simulink model "Aruduino_DCmoter_test"  (R2015a)
settings: Solver=ode3  StartTime=0.0  StopTime=10.0  RelTol=1e-3
libraries: arduinolib x5
settings Model: SimulationMode=external  ExtModeTrigDuration=2  Creator=Edwin Ri  LastModifiedBy=Edwin Ri
settings OptimizationCC: OptimizeModelRefInitCode=on  LifeSpan=1
settings DebuggingCC: UnderspecifiedInitializationDetection=Classic  MergeDetectMultiDrivingBlocksExec=none
settings HardwareCC: ProdBitPerInt=16  ProdBitPerPointer=8  ProdIntDivRoundTo=Zero  ProdEndianess=LittleEndian  ProdWordSize=8  ProdHWDeviceType=Atmel->AVR
settings RTWCC: SystemTargetFile=realtime.tlc  GenerateMakefile=off  TemplateMakefile=realtime.tmf  Description=Run on Target Hardware  RTWVerbose=off
settings ERTTargetCC: CombineOutputUpdateFcns=off  ExtMode=on  ExtModeTransport=3  ExtModeMexArgs=0 4 115200 5  ERTSrcFileBannerTemplate=realtime_code_template.cgt  ERTHdrFileBannerTemplate=realtime_code_template.cgt  ERTDataSrcFileTemplate=realtime_code_template.cgt  ERTDataHdrFileTemplate=realtime_code_template.cgt  ERTCustomFileTemplate=realtime_file_process.tlc

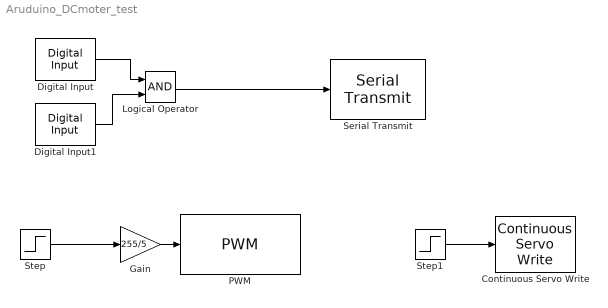
== system Aruduino_DCmoter_test ==
  Continuous Servo Write : arduinolib/Continuous Servo Write  pinNumber=5  blockPlatform=arduino
  Digital Input : arduinolib/Digital Input  pinNumber=2  sampleTime=1  blockPlatform=arduino
  Digital Input1 : arduinolib/Digital Input  pinNumber=3  sampleTime=1  blockPlatform=arduino
  Gain : Gain  Gain=255/5
  Logical Operator : Logic  AllPortsSameDT=off  OutDataTypeStr=boolean
  PWM : arduinolib/PWM  pinNumber=11  blockPlatform=arduino
  Serial Transmit : arduinolib/Serial Transmit  portNumber=0  blockPlatform=arduino
  Step : Step  Time=8  Before=2  After=0  SampleTime=0
  Step1 : Step  Time=8  Before=30  After=0  SampleTime=0
  wires:
  Gain/1 -> PWM/1
  Step/1 -> Gain/1
  Step1/1 -> Continuous Servo Write/1
  Digital Input/1 -> Logical Operator/1
  Digital Input1/1 -> Logical Operator/2
  Logical Operator/1 -> Serial Transmit/1
